simulink model "AMCFOC"  (R2023b)
settings: Solver=FixedStepDiscrete  StartTime=0.0  StopTime=10.0  RelTol=1e-3  EnableMultiTasking=on
undefined symbols (not defined in the file): D1, D2, D3, D4, P
settings Model: DataDictionary=amcfoc.sldd  Creator=mfussi  LastModifiedBy=mfussi
settings SolverCC: ConcurrentTasks=on
settings OptimizationCC: DefaultParameterBehavior=Inlined  UseDivisionForNetSlopeComputation=on  DefaultUnderspecifiedDataType=single  EnhancedBackFolding=on  ZeroExternalMemoryAtStartup=off  ZeroInternalMemoryAtStartup=off  OptimizeBlockOrder=speed  DifferentSizesBufferReuse=on  OptimizationCustomize=off  EfficientTunableParamExpr=on
settings DebuggingCC: ParameterTunabilityLossMsg=error
settings HardwareCC: ProdBitPerPointer=32  ProdBitPerSizeT=32  ProdBitPerPtrDiffT=32  ProdLargestAtomicInteger=Long  ProdLargestAtomicFloat=Double  ProdWordSize=32  ProdHWDeviceType=ARM Compatible->ARM Cortex-M
settings SFSimCC: MATLABDynamicMemAlloc=off
settings RTWCC: Description=Embedded Coder  SystemTargetFile=ert.tlc  GenCodeOnly=on  PackageGeneratedCodeAndArtifacts=on  TemplateMakefile=ert_default_tmf  Toolchain=GNU Tools for ARM Embedded Processors  BuildConfiguration=Faster Runs
settings CodeAppCC: ForceParamTrailComments=on  IgnoreCustomStorageClasses=off  OperatorAnnotations=on  SimulinkDataObjDesc=on  SFDataObjDesc=on  InsertBlockDesc=on
settings ERTTargetCC: TargetLangStandard=C99 (ISO)  CodeReplacementLibrary=ARM Cortex-M,iCubTech  GenerateSampleERTMain=on  SupportNonFinite=off  SupportComplex=off  InlinedParameterPlacement=NonHierarchical  ERTCustomFileTemplate=example_file_process.tlc

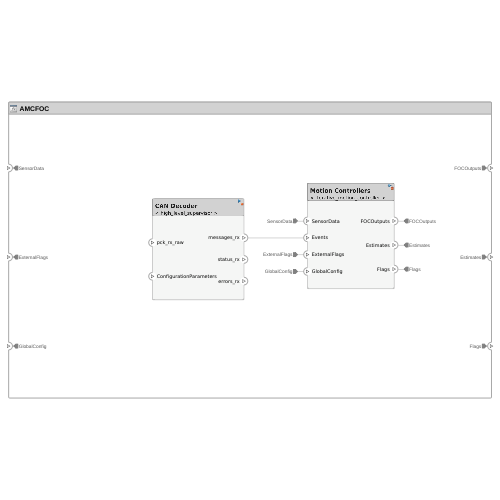
[thumbnail: Simulink's stored preview of the top-level diagram]
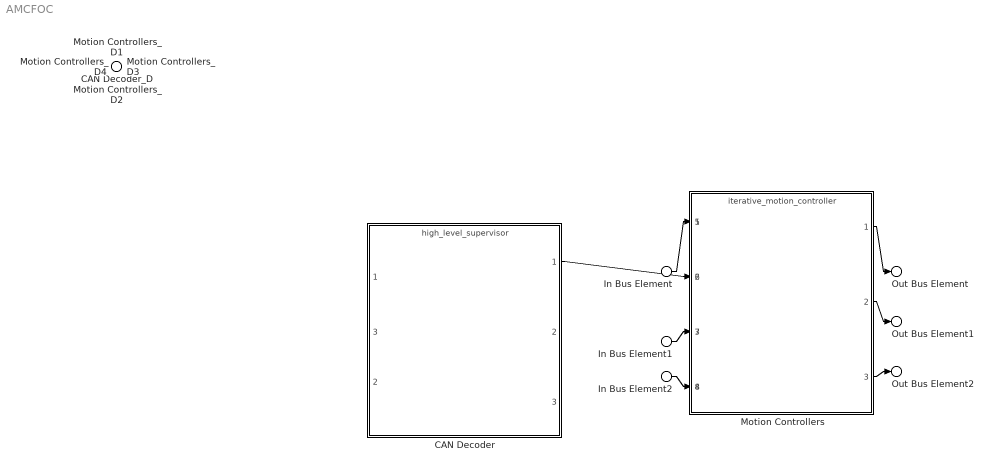
== system AMCFOC ==
  In Bus Element : Inport  PortName=SensorData
  In Bus Element1 : Inport  Port=2  PortName=ExternalFlags
  In Bus Element2 : Inport  Port=3  PortName=GlobalConfig
  CAN Decoder_D : Inport  Port=4  OutputFunctionCall=on
  Motion Controllers_D1 : Inport  Port=5  OutputFunctionCall=on
  Motion Controllers_D2 : Inport  Port=6  OutputFunctionCall=on
  Motion Controllers_D3 : Inport  Port=7  OutputFunctionCall=on
  Motion Controllers_D4 : Inport  Port=8  OutputFunctionCall=on
  CAN Decoder : ModelReference  ModelNameDialog=high_level_supervisor  SimulationMode=Normal  ScheduleRates=on  ModelEventPortInfo=P:D1[-2][0][0]  ModelReferenceVersion=1.3
      settings: PortSchema="{\"entries\":[{\"content\":{\"headerSize\":38,\"margin\":15,\"minimumSpacing\":25,\"sides\":[{\"content\":{\"connectorIds\":[\"In1\",\"In2\"]},\"type\":\"ConnectorPlacement.EquallySpacedRectSide\",\"uuid\":\"ad9e16c1-53b5-404c-89e4-025a25695e1a\"},{\"content\":{\"connectorIds\":[\"Out1\",\"Out2\",\"Out3\"],\"side\":\"RIGHT\"},\"type\":\"ConnectorPlacement.EquallySpacedRectSide\",\"uuid\":\"ffa85564-4044-494a-a694-0f3690d98b5d\"},{\"content\":{\"side\":\"TOP\"},\"type\":\"ConnectorPlacement.EquallySpacedRectSide\",\"uuid\":\"c7160a56-fbc7-4ea5-b3fd-3e2829dcdab4\"},{\"content\":{\"connectorIds\":[\"In3\"],\"side\":\"HIDDEN\"},\"type\":\"ConnectorPlacement.EquallySpacedRectSide\",\"uuid\":\"263c822e-8129-41e7-9458-192b6196c12c\"}]},\"type\":\"ConnectorPlacement.EquallySpacedConnector\",\"uuid\":\"f1c79445-b86c-4247-bb75-1a126bddf195\"}],\"packageUris\":[\"http://schema.mathworks.com/mf0/Connector/R2020b\"],\"version\":\"1.0\"}"
  Motion Controllers : ModelReference  ModelNameDialog=iterative_motion_controller.slx  SimulationMode=Normal  ScheduleRates=on  CachedPortDiscreteRates=[1.1428571428571438E-6;3.65714285714286E-5;0.001;0.01]  ModelEventPortInfo=P:D1[1.1428571428571438E-6][0][0],P:D2[3.65714285714286E-5][0][0],P:D3[0.001][0][0],P:D4[0.01][0][0]  ModelReferenceVersion=1.101
      settings: PortSchema="{\"entries\":[{\"content\":{\"headerSize\":38,\"margin\":15,\"minimumSpacing\":25,\"sides\":[{\"content\":{\"connectorIds\":[\"In1\",\"In2\",\"In3\",\"In4\"]},\"type\":\"ConnectorPlacement.EquallySpacedRectSide\",\"uuid\":\"8eda670a-b8e9-4980-b06b-e5352b47324e\"},{\"content\":{\"connectorIds\":[\"Out1\",\"Out2\",\"Out3\"],\"side\":\"RIGHT\"},\"type\":\"ConnectorPlacement.EquallySpacedRectSide\",\"uuid\":\"79db1cad-a499-4fde-a889-975af68c44fc\"},{\"content\":{\"side\":\"TOP\"},\"type\":\"ConnectorPlacement.EquallySpacedRectSide\",\"uuid\":\"390fb433-bff9-464b-a3b6-d8b4ca75b5ba\"},{\"content\":{\"connectorIds\":[\"In5\",\"In6\",\"In7\",\"In8\"],\"side\":\"HIDDEN\"},\"type\":\"ConnectorPlacement.EquallySpacedRectSide\",\"uuid\":\"1ed1d734-2936-4467-9da5-f2554daa4cea\"}]},\"type\":\"ConnectorPlacement.EquallySpacedConnector\",\"uuid\":\"36d8834e-6601-4a2a-af9e-11089dfdbeb5\"}],\"packageUris\":[\"http://schema.mathworks.com/mf0/Connector/R2020b\"],\"version\":\"1.0\"}"
  Out Bus Element : Outport  PortName=FOCOutputs
  Out Bus Element1 : Outport  Port=2  PortName=Estimates
  Out Bus Element2 : Outport  Port=3  PortName=Flags
  wires:
  In Bus Element/1 -> Motion Controllers/1
  In Bus Element1/1 -> Motion Controllers/3
  In Bus Element2/1 -> Motion Controllers/4
  Motion Controllers/1 -> Out Bus Element/1
  Motion Controllers/2 -> Out Bus Element1/1
  Motion Controllers/3 -> Out Bus Element2/1
  CAN Decoder/1 -> Motion Controllers/2
